simulink model "Buck_Converter_Modelling"  (R2015a)
settings: Solver=ode45  StartTime=0.0  StopTime=0.01  RelTol=1e-3
values from neighbouring files (symbols this model uses):
  C = 19.5e-06    (= 1.95e-05)    [Buck_Converter_Modelling_Script.m]
  D = 0.416    [Buck_Converter_Modelling_Script.m]
  Fsw = 400e03    (= 400000)    [Buck_Converter_Modelling_Script.m]
  L = 12.12e-06    (= 1.212e-05)    [Buck_Converter_Modelling_Script.m]
  R = 5    [Buck_Converter_Modelling_Script.m]
  Vin = 12    [Buck_Converter_Modelling_Script.m]
settings Model: Creator=Koustubh  LastModifiedBy=Koustubh

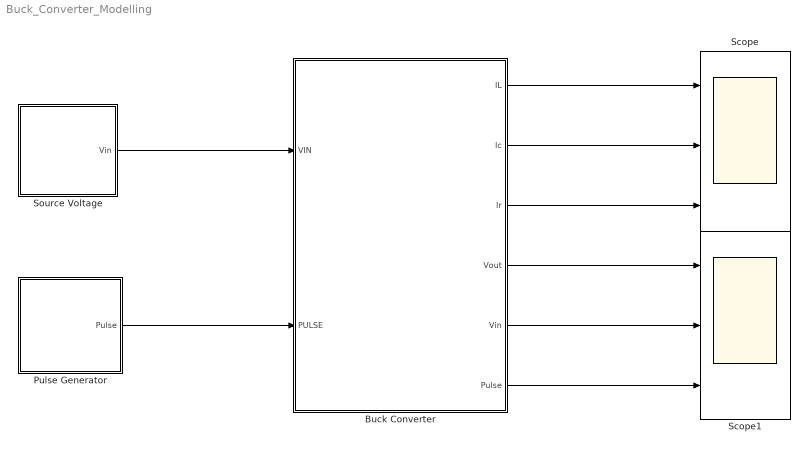
== system Buck_Converter_Modelling ==
  Buck Converter : Subsystem  TreatAsAtomicUnit=on
  Pulse Generator : Subsystem  TreatAsAtomicUnit=on
  Scope : Scope  NumInputPorts=3
      settings: YMin=-5~-5~-5  YMax=5~5~5
  Scope1 : Scope  NumInputPorts=3
      settings: YMin=-5~-5~-5  YMax=5~5~5
  Source Voltage : Subsystem  TreatAsAtomicUnit=on
  wires:
  Pulse Generator/1(Pulse) -> Buck Converter/2(PULSE)
  Source Voltage/1(Vin) -> Buck Converter/1(VIN)
  Buck Converter/1(IL) -> Scope/1
  Buck Converter/2(Ic) -> Scope/2
  Buck Converter/4(Vout) -> Scope1/1
  Buck Converter/5(Vin) -> Scope1/2
  Buck Converter/6(Pulse) -> Scope1/3
  Buck Converter/3(Ir) -> Scope/3

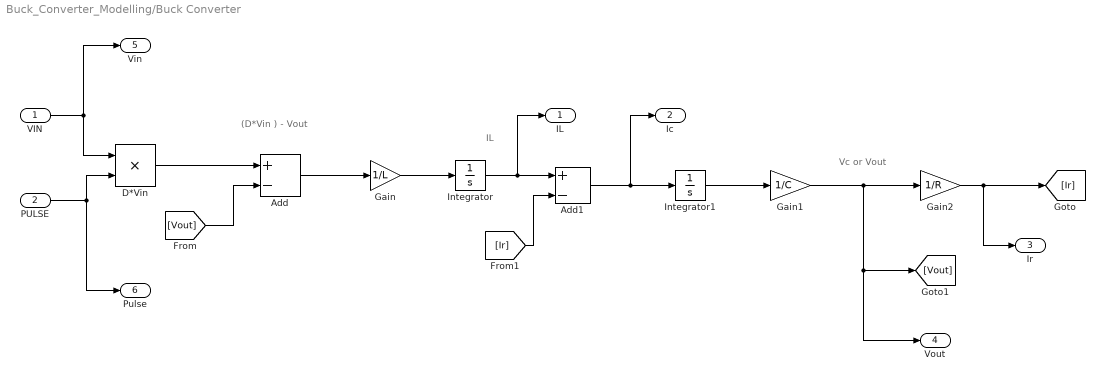
== system Buck_Converter_Modelling/Buck Converter ==
  note: Vc or Vout
  note: IL
  note: (D*Vin ) - Vout
  VIN : Inport
  PULSE : Inport  Port=2
  Add : Sum  Inputs=+-
  Add1 : Sum  Inputs=+-
  D*Vin : Product
  Gain : Gain  Gain=1/L
  Gain1 : Gain  Gain=1/C
  Gain2 : Gain  Gain=1/R
  Integrator : Integrator
  Integrator1 : Integrator
  IL : Outport
  Ic : Outport  Port=2
  Ir : Outport  Port=3
  Vout : Outport  Port=4
  Vin : Outport  Port=5
  Pulse : Outport  Port=6
  wires:
  VIN/1 -> Vin/1, D*Vin/1
  PULSE/1 -> Pulse/1, D*Vin/2
  D*Vin/1 -> Add/1
  [Vout] -> Add/2
  Add/1 -> Gain/1
  Gain/1 -> Integrator/1
  Integrator/1 -> IL/1, Add1/1
  [Ir] -> Add1/2
  Add1/1 -> Ic/1, Integrator1/1
  Integrator1/1 -> Gain1/1
  Gain1/1 -> Vout/1, [Vout], Gain2/1
  Gain2/1 -> [Ir], Ir/1

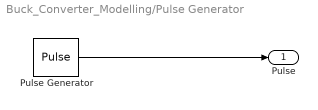
== system Buck_Converter_Modelling/Pulse Generator ==
  Pulse Generator : DiscretePulseGenerator  PulseType=Time based  Period=1/Fsw  PulseWidth=D*100
  Pulse : Outport
  wires:
  Pulse Generator/1 -> Pulse/1

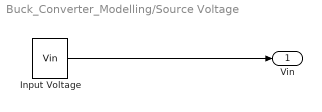
== system Buck_Converter_Modelling/Source Voltage ==
  Input Voltage : Constant  Value=Vin
  Vin : Outport
  wires:
  Input Voltage/1 -> Vin/1
